simulink model "Helicopter_SetPoint_eInt_real"  (R2018a)
settings: Solver=ode4  StartTime=0.0  StopTime=inf  FixedStep=0.2  RelTol=1e-3
values from neighbouring files (symbols this model uses):
  Ad = sys_d.a    [Helicopter_Values.m]
  Bd = sys_d.b    [Helicopter_Values.m]
  Cd = sys_d.c    [Helicopter_Values.m]
  p_r_op = -10*pi/180    (= -0.174532925199)    [Helicopter_Values.m]
  Vmp_op = (kyy*mheli*g*cos(p_r_op)*lcm)/(kyy*kpp -kyp*kpy)    [Helicopter_Values.m]
  Vmy_op = kyp*Vmp_op/kyy    [Helicopter_Values.m]
  wp_op = 0    [Helicopter_Values.m]
  wy_op = 0    [Helicopter_Values.m]
  y_r_op = pi/2    (= 1.57079632679)    [Helicopter_Values.m]
undefined symbols (not defined in the file or in its folder): daq, K, k_lqr_e
libraries: daqlib x2, realtime_pacer_lib x1
settings Model: Creator=pacoa  LastModifiedBy=pacoa

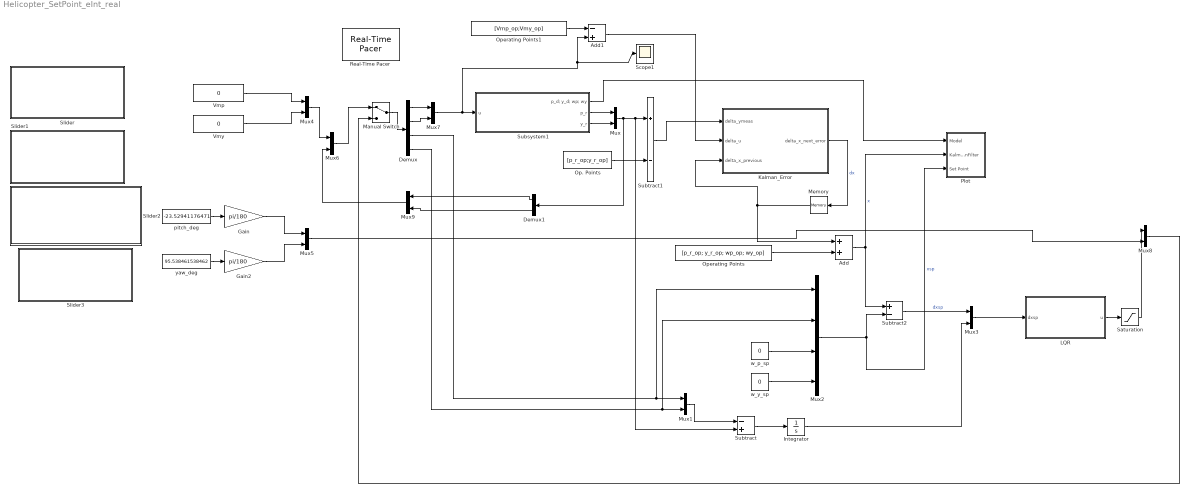
== system Helicopter_SetPoint_eInt_real ==
  Add : Sum
  Add1 : Sum  Inputs=-+
  Demux : Demux
  Demux1 : Demux  Outputs=2
  Gain : Gain  Gain=pi/180
  Gain2 : Gain  Gain=pi/180
  Integrator : Integrator  InitialCondition=[0;0]
  Kalman_Error : MATLAB Function  TreatAsAtomicUnit=on
  LQR : Subsystem
  Manual Switch : ManualSwitch
  Memory : Memory  InitialCondition=[0;0;0;0]
  Mux{,1,3..9} (9 alike) : Mux  Inputs=2
  Mux2 : Mux
  Op. Points : Constant  Value=[p_r_op;y_r_op]
  Operating Points : Constant  Value=[p_r_op; y_r_op; wp_op; wy_op]
  Operating Points1 : Constant  Value=[Vmp_op;Vmy_op]
  Plot : Subsystem
  Real-Time Pacer : realtime_pacer_lib/Real-Time Pacer  simTimePerRealTime=1
  Saturation : Saturate  UpperLimit=[3;3]  LowerLimit=[0;0]
  Scope1 : Scope
  Slider : Subsystem  DialogController=hmiCreateDDGDialog  IsWebBlock=on  mask(MWDashboardBlock){webBlockId=04463d73-d6a9-4b3d-abfe-2f563ab264e6, webBlockType=slider, ShowInLibBrowser=on, ShowInitialText=on, HMISrcModelName=Helicopter_SetPoint_eInt_real}
      mask prompts: webBlockId "WebBlock Id"; webBlockType "WebBlock Type"; HMISrcModelName "Source Model"
      mask help: SimulinkHMI:dialogs:SliderDialogDesc
      mask Help: helpview([docroot '/mapfiles/simulink.map'], 'hmi_slider')
      mask Display:
      | if strcmp(get_param(bdroot(gcb),'BlockDiagramType'), 'library')
      |     image([(matlabroot) '/toolbox/simulink/hmi/icons/Slider.png']);
      | end
  Slider1 : Subsystem  DialogController=hmiCreateDDGDialog  IsWebBlock=on  mask(MWDashboardBlock){webBlockId=82fec370-2a65-419d-b4f2-61c4ae5ab55a, webBlockType=slider, ShowInLibBrowser=on, ShowInitialText=on, HMISrcModelName=Helicopter_SetPoint_eInt_real}
      mask prompts: webBlockId "WebBlock Id"; webBlockType "WebBlock Type"; HMISrcModelName "Source Model"
      mask help: SimulinkHMI:dialogs:SliderDialogDesc
      mask Help: helpview([docroot '/mapfiles/simulink.map'], 'hmi_slider')
      mask Display:
      | if strcmp(get_param(bdroot(gcb),'BlockDiagramType'), 'library')
      |     image([(matlabroot) '/toolbox/simulink/hmi/icons/Slider.png']);
      | end
  Slider2 : Subsystem  DialogController=hmiCreateDDGDialog  IsWebBlock=on  mask(MWDashboardBlock){webBlockId=4346c81c-e5d4-41da-88ba-4ceee90b391b, webBlockType=slider, ShowInLibBrowser=on, ShowInitialText=on, HMISrcModelName=Helicopter_SetPoint_eInt_real}
      mask prompts: webBlockId "WebBlock Id"; webBlockType "WebBlock Type"; HMISrcModelName "Source Model"
      mask help: SimulinkHMI:dialogs:SliderDialogDesc
      mask Help: helpview([docroot '/mapfiles/simulink.map'], 'hmi_slider')
      mask Display:
      | if strcmp(get_param(bdroot(gcb),'BlockDiagramType'), 'library')
      |     image([(matlabroot) '/toolbox/simulink/hmi/icons/Slider.png']);
      | end
  Slider3 : Subsystem  DialogController=hmiCreateDDGDialog  IsWebBlock=on  mask(MWDashboardBlock){webBlockId=44ebcc4a-aa43-4d83-9862-a30861b04c6c, webBlockType=slider, ShowInLibBrowser=on, ShowInitialText=on, HMISrcModelName=Helicopter_SetPoint_eInt_real}
      mask prompts: webBlockId "WebBlock Id"; webBlockType "WebBlock Type"; HMISrcModelName "Source Model"
      mask help: SimulinkHMI:dialogs:SliderDialogDesc
      mask Help: helpview([docroot '/mapfiles/simulink.map'], 'hmi_slider')
      mask Display:
      | if strcmp(get_param(bdroot(gcb),'BlockDiagramType'), 'library')
      |     image([(matlabroot) '/toolbox/simulink/hmi/icons/Slider.png']);
      | end
  Subsystem1 : Subsystem
  Subtract : Sum  Inputs=-+
  Subtract1 : Sum  Inputs=+-
  Subtract2 : Sum  Inputs=+-
  Vmp : Constant  Value=0
  Vmy : Constant  Value=0
  pitch_deg : Constant  Value=-23.52941176471
  w_p_sp : Constant  Value=0
  w_y_sp : Constant  Value=0
  yaw_deg : Constant  Value=95.538461538462
  wires:
  Add1/1 -> Kalman_Error/2(delta_u)
  Subtract2/1 -> Mux3/1  "dxsp"
  Integrator/1 -> Mux3/2
  Mux3/1 -> LQR/1(dxsp)
  Subtract1/1 -> Kalman_Error/1(delta_ymeas)
  Gain/1 -> Mux5/1
  w_p_sp/1 -> Mux2/3
  Mux/1 -> Demux1/1, Subtract/2, Subtract1/1
  Subsystem1/1(p_d; y_d; wp; wy) -> Plot/1(Model)
  Gain2/1 -> Mux5/2
  Kalman_Error/1(delta_x_next_error) -> Memory/1  "dx"
  Subtract/1 -> Integrator/1
  Add/1 -> Subtract2/1, Plot/2(KalmanFilter)  "x"
  Subsystem1/3(y_r) -> Mux/2
  w_y_sp/1 -> Mux2/4
  Op. Points/1 -> Subtract1/2
  Mux2/1 -> Subtract2/2, Plot/3(Set Point)  "xsp"
  Subsystem1/2(p_r) -> Mux/1
  Operating Points/1 -> Add/2
  Mux1/1 -> Subtract/1
  LQR/1(u) -> Saturation/1
  Vmp/1 -> Mux4/1
  Vmy/1 -> Mux4/2
  Operating Points1/1 -> Add1/1
  pitch_deg/1 -> Gain/1
  yaw_deg/1 -> Gain2/1
  Memory/1 -> Add/1, Kalman_Error/3(delta_x_previous)
  Mux6/1 -> Manual Switch/1
  Mux4/1 -> Mux6/1
  Manual Switch/1 -> Demux/1
  Demux/1 -> Mux7/1
  Demux/2 -> Mux7/2
  Mux7/1 -> Scope1/1, Add1/2, Subsystem1/1(u)
  Demux/3 -> Mux2/1, Mux1/1
  Demux/4 -> Mux2/2, Mux1/2
  Saturation/1 -> Mux8/1
  Demux1/1 -> Mux9/1
  Demux1/2 -> Mux9/2
  Mux8/1 -> Manual Switch/2
  Mux5/1 -> Mux8/2
  Mux9/1 -> Mux6/2

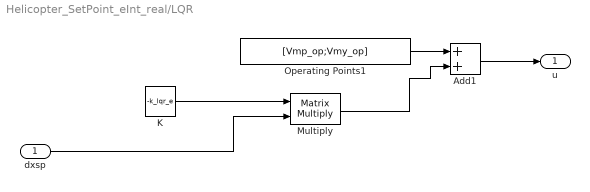
== system Helicopter_SetPoint_eInt_real/LQR ==
  dxsp : Inport
  Add1 : Sum
  K : Constant  Value=-k_lqr_e
  Multiply : Product  Multiplication=Matrix(*)
  Operating Points1 : Constant  Value=[Vmp_op;Vmy_op]
  u : Outport
  wires:
  K/1 -> Multiply/1
  Multiply/1 -> Add1/2
  dxsp/1 -> Multiply/2
  Operating Points1/1 -> Add1/1
  Add1/1 -> u/1

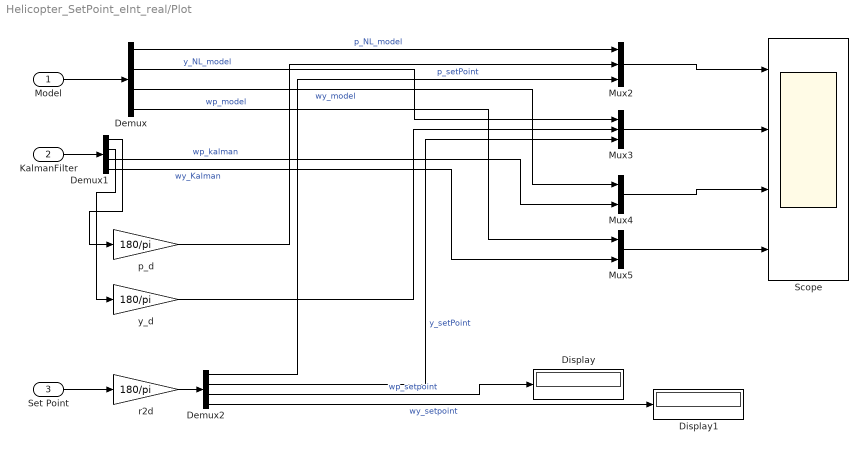
== system Helicopter_SetPoint_eInt_real/Plot ==
  Model : Inport
  KalmanFilter : Inport  Port=2
  Set Point : Inport  Port=3
  Demux : Demux
  Demux1 : Demux
  Demux2 : Demux
  Display : Display
  Display1 : Display
  Mux2 : Mux  Inputs=3
  Mux3 : Mux  Inputs=3
  Mux4 : Mux  Inputs=2
  Mux5 : Mux  Inputs=2
  Scope : Scope  NumInputPorts=4
  p_d : Gain  Gain=180/pi
  r2d : Gain  Gain=180/pi
  y_d : Gain  Gain=180/pi
  wires:
  KalmanFilter/1 -> Demux1/1
  Mux2/1 -> Scope/1
  Demux/3 -> Mux4/1  "wy_model"
  Demux1/4 -> Mux5/2  "wy_Kalman"
  Mux4/1 -> Scope/3
  Demux1/3 -> Mux4/2  "wp_kalman"
  Demux/1 -> Mux2/1  "p_NL_model"
  Demux/4 -> Mux5/1  "wp_model"
  Mux3/1 -> Scope/2
  p_d/1 -> Mux2/2
  Mux5/1 -> Scope/4
  Demux1/1 -> p_d/1
  y_d/1 -> Mux3/2
  Demux/2 -> Mux3/1  "y_NL_model"
  Demux1/2 -> y_d/1
  Model/1 -> Demux/1
  Set Point/1 -> r2d/1
  r2d/1 -> Demux2/1
  Demux2/1 -> Mux2/3  "p_setPoint"
  Demux2/2 -> Mux3/3  "y_setPoint"
  Demux2/3 -> Display/1  "wp_setpoint"
  Demux2/4 -> Display1/1  "wy_setpoint"

== system Helicopter_SetPoint_eInt_real/Slider ==

== system Helicopter_SetPoint_eInt_real/Slider1 ==

== system Helicopter_SetPoint_eInt_real/Slider2 ==

== system Helicopter_SetPoint_eInt_real/Slider3 ==

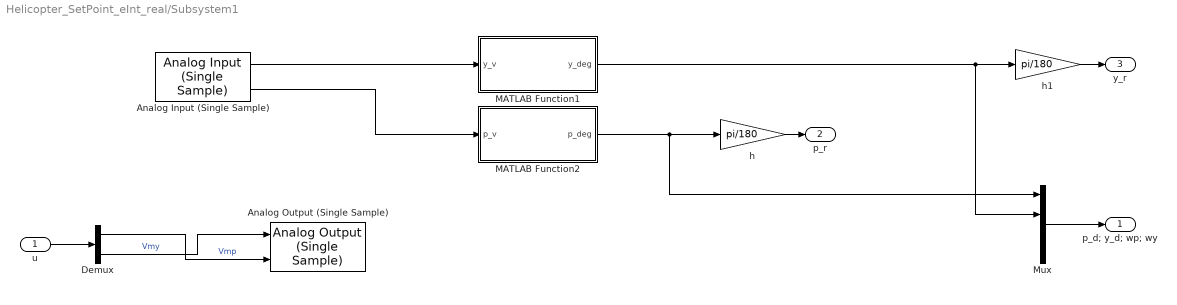
== system Helicopter_SetPoint_eInt_real/Subsystem1 ==
  u : Inport
  Analog Input (Single Sample) : daqlib/Analog Input (Single Sample)  DeviceMenu=ni Dev5 (USB-6001)  Device=ni Dev5 (USB-6001)  ObjConstructor=daq.createSession('ni')  BlockSampleTime=0.2  NChannelsSelected=2  Channels=1$ai0$$Dev5$1$1$2$1$#1$ai1$$Dev5$1$1$2$1$#0$ai2$$Dev5$1$1$2$1$#0$ai3$$Dev5$1$1$2$1$#0$ai4$$Dev5$1$1$1$1$#0$ai5$$Dev5$1$1$1$1$#0$ai6$$Dev5$1$1$1$1$#0$ai7$$Dev5$1$1$1$1$#  NPorts=1 per channel  OutputTimestamp=off
      settings: SourceProductName=Data Acquisition Toolbox  SourceProductBaseCode=DA
  Analog Output (Single Sample) : daqlib/Analog Output (Single Sample)  DeviceMenu=ni Dev5 (USB-6001)  Device=ni Dev5 (USB-6001)  ObjConstructor=daq.createSession('ni')  NChannelsSelected=2  Channels=1$ao0$$Dev5$1$1$N/A$#1$ao1$$Dev5$1$1$N/A$#  NPorts=1 per channel  BlockSampleTime=0.2
      settings: SourceProductName=Data Acquisition Toolbox  SourceProductBaseCode=DA
  Demux : Demux  Outputs=2
  MATLAB Function1 : MATLAB Function  TreatAsAtomicUnit=on
  MATLAB Function2 : MATLAB Function  TreatAsAtomicUnit=on
  Mux : Mux
  h : Gain  Gain=pi/180
  h1 : Gain  Gain=pi/180
  p_d; y_d; wp; wy : Outport  PortDimensions=[4 1]
  p_r : Outport  Port=2  PortDimensions=1
  y_r : Outport  Port=3  PortDimensions=1
  wires:
  Mux/1 -> p_d; y_d; wp; wy/1
  h/1 -> p_r/1
  u/1 -> Demux/1
  Demux/1 -> Analog Output (Single Sample)/2  "Vmp"
  Demux/2 -> Analog Output (Single Sample)/1  "Vmy"
  Analog Input (Single Sample)/2 -> MATLAB Function2/1(p_v)
  Analog Input (Single Sample)/1 -> MATLAB Function1/1(y_v)
  MATLAB Function2/1(p_deg) -> h/1, Mux/1
  MATLAB Function1/1(y_deg) -> h1/1, Mux/2
  h1/1 -> y_r/1

== matlab function Helicopter_SetPoint_eInt_real/Subsystem1/MATLAB Function1 ==
  data: y_v input size=[1]; y_deg output size=[1]
function y_deg = y_V_to_deg(y_v)
error = 0.19;
%error = 0;
y_v = y_v -error;
V_max = 5;
V_min = 0;
deg_max = 180;
deg_min = 0;
m =(deg_max - deg_min)/(V_max - V_min)
y_deg = m*(y_v -V_min) + deg_min;

== matlab function Helicopter_SetPoint_eInt_real/Kalman_Error ==
  data: delta_ymeas input; delta_x_next_error output; delta_u input; delta_x_previous input; K parameter; Ad parameter; Bd parameter; Cd parameter
function delta_x_next_error = mykalman_error(delta_ymeas,delta_u,delta_x_previous, K, Ad, Bd, Cd)

delta_x_next_error = Ad*delta_x_previous +Bd*delta_u +K*(delta_ymeas -Cd*delta_x_previous);

== matlab function Helicopter_SetPoint_eInt_real/Subsystem1/MATLAB Function2 ==
  data: p_v input size=[1]; p_deg output size=[1]
function p_deg = p_V_to_deg(p_v)
error = 0.22;
%error = 0;
p_v = p_v - error;
V_max = 5;
V_min = 0;
deg_max = 45;
deg_min = -45;
m =(deg_max - deg_min)/(V_max - V_min)
p_deg = m*(p_v -V_min) + deg_min;
